simulink model "mtv1_with_slosh_with_valve_delay"  (R2014b)
settings: Solver=ode4  SolverMode=SingleTasking  StartTime=0.0  StopTime=sim_stop_time  FixedStep=sim_time_step_size  RelTol=1e-3
PreLoadFcn:
  | nimbus_bus_all;
  | mtv_bus_all;
undefined symbols (not defined in the file or in its folder): csc_cnt_attitude_control, csc_cnt_attitude_control_lib, csc_cnt_dt, csc_egt_egc_thruster, csc_egt_egc_thruster_lib, csc_eom_six_dof_integration_fwdeuler, csc_eom_six_dof_integration_lib, csc_ppc_phase_plane_ctrl, csc_ppc_phase_plane_ctrl_lib, csc_rigid_body_dynamics, csc_rigid_body_dynamics_lib, csc_sim_mtv_simulation, csc_sim_mtv_simulation_lib, csc_thl_thrusters_mtv, csc_thl_thrusters_mtv_lib, csci_fsw_mtv, csci_fsw_mtv_lib, csci_gsse_mtv, csci_gsse_mtv_lib, csu_rrk_rotational_kinematics, csu_rrk_rotational_kinematics_lib, csu_rtk_translational_kinematics, csu_rtk_translational_kinematics_lib, csu_tpl_thruster_propellant_mtv, csu_tpl_thruster_propellant_mtv_lib, egt_feed_pressure, egt_g_times_isp, egt_pc_to_thrust_offset, egt_pc_to_thrust_slope, gdn_altitude_transition_free_drift_landing, gdn_altitude_transition_free_drift_takeoff, ini_epoch_seconds, ini_landed_flag, ini_thrust_to_weight_takeoff_limit, mpl_gn2_mass_initial, mpl_htp_mass_initial, ppc_coarse_thr_delay, ppc_fine_thr_delay, sim_time_step_size, swm_num_switches, tpl_coarse_acs_thrust_to_isp, tpl_egc_chamber_pressure_to_thrust, tpl_egc_throttle_to_mdot_gain, tpl_egc_throttle_to_thrust, tpl_egc_throttle_to_thrust_gain
libraries: util_common_lib x17, util_info_lib x13, util_quat_lib x8, simulink x8, csu_spv_simulated_press_valves_lib x4, csu_cfe_cfe_time_lib x2, csu_tlm_telemetry_lib x2, util_event_lib x2, util_frame_rotation_lib x2, csc_act_actuator_manager_mtv_lib x1, csc_cmp_command_mode_process_mtv_lib x1, util_extra_lib x1
(part 1 of 2)
settings Model: ExtModeTrigDuration=100  Creator=ianmga  LastModifiedBy=mstewart
settings DataIOCC: LimitDataPoints=off  SaveOutput=off  SaveTime=off  StateSaveName=tmp_raccel_xout  SignalLoggingName=raw_event_logs
settings OptimizationCC: ExpressionDepthLimit=2147483647  InitFltsAndDblsToZero=on  OptimizeModelRefInitCode=on
settings DebuggingCC: CheckSSInitialOutputMsg=off  UnderspecifiedInitializationDetection=Classic  MergeDetectMultiDrivingBlocksExec=none  UnderSpecifiedDataTypeMsg=warning  FcnCallInpInsideContextMsg=UseLocalSettings  BusObjectLabelMismatch=error  StateNameClashWarn=warning  StrictBusMsg=WarnOnBusTreatedAsVector
settings HardwareCC: TargetHWDeviceType=32-bit Generic
settings SFSimCC: SimParseCustomCode=off
settings SFSimCC: SimUserIncludeDirs=|
  | ../sim/fhw/sensors/cameras/kir
  | ../fsw/est/kcv
  | ../fsw/est/kfd
  | ../externals/minopencv/include
settings RTWCC: SystemTargetFile=ert.tlc  GenCodeOnly=on  TemplateMakefile=ert_default_tmf  Description=Embedded Coder  RetainRTWFile=on  ProcessScript=ert_make_rtw_hook  RTWUseSimCustomCode=on
settings RTWCC: CustomInclude=|
  | ../sim/fhw/sensors/cameras/kir
  | ../fsw/est/kcv
  | ../fsw/est/kfd
  | ../externals/minopencv/include
settings CodeAppCC: ForceParamTrailComments=on  IgnoreCustomStorageClasses=off  MaxIdLength=128  SimulinkDataObjDesc=on  SFDataObjDesc=on  MangleLength=10  CustomSymbolStrType=$N$R$M  InsertBlockDesc=on  InternalIdentifier=Classic  ReqsInCode=on
settings ERTTargetCC: GenerateSampleERTMain=on  MultiInstanceERTCode=on  CodeInterfacePackaging=Reusable function  RootIOFormat=Structure reference  ERTCustomFileTemplate=csl_interface.tlc

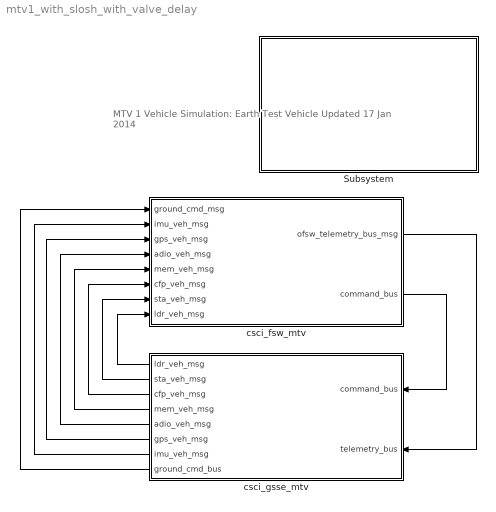
== system mtv1_with_slosh_with_valve_delay ==
  note: MTV 1 Vehicle Simulation: Earth Test Vehicle
      |
      | Updated 17 Jan 2014
  Subsystem : Subsystem
      mask Display: image('nimbus2.png')
  csci_fsw_mtv : Subsystem  AncestorBlock=csci_fsw_mtv_lib/csci_fsw_mtv
  csci_gsse_mtv : Subsystem  AncestorBlock=csci_gsse_mtv_lib/csci_gsse_mtv
  wires:
  csci_fsw_mtv/1(ofsw_telemetry_bus_msg) -> csci_gsse_mtv/2(telemetry_bus)
  csci_gsse_mtv/2(sta_veh_msg) -> csci_fsw_mtv/7(sta_veh_msg)
  csci_fsw_mtv/2(command_bus) -> csci_gsse_mtv/1(command_bus)
  csci_gsse_mtv/1(ldr_veh_msg) -> csci_fsw_mtv/8(ldr_veh_msg)
  csci_gsse_mtv/3(cfp_veh_msg) -> csci_fsw_mtv/6(cfp_veh_msg)
  csci_gsse_mtv/4(mem_veh_msg) -> csci_fsw_mtv/5(mem_veh_msg)
  csci_gsse_mtv/5(adio_veh_msg) -> csci_fsw_mtv/4(adio_veh_msg)
  csci_gsse_mtv/6(gps_veh_msg) -> csci_fsw_mtv/3(gps_veh_msg)
  csci_gsse_mtv/8(ground_cmd_bus) -> csci_fsw_mtv/1(ground_cmd_msg)
  csci_gsse_mtv/7(imu_veh_msg) -> csci_fsw_mtv/2(imu_veh_msg)

== system mtv1_with_slosh_with_valve_delay/Subsystem ==

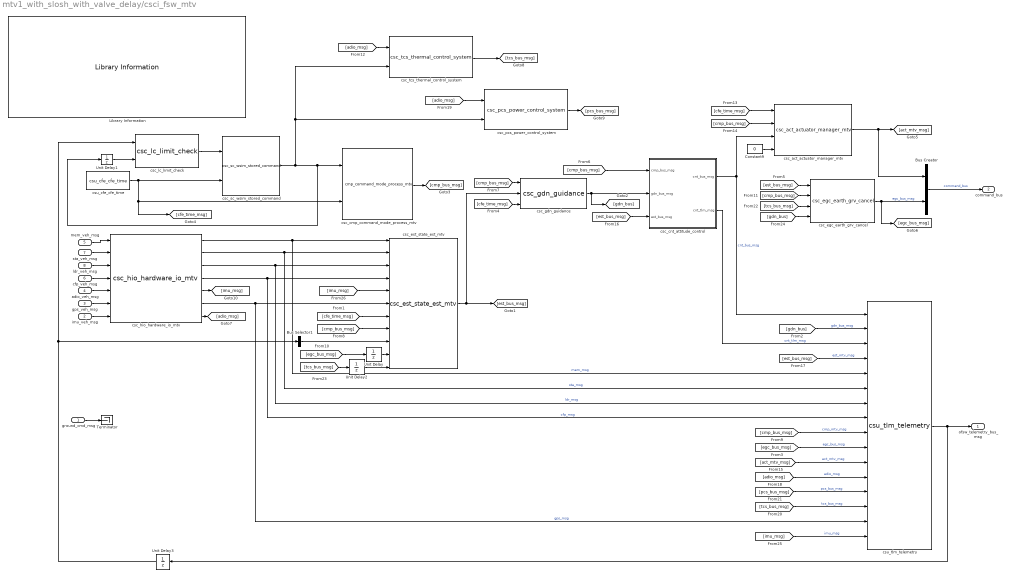
== system mtv1_with_slosh_with_valve_delay/csci_fsw_mtv ==
  ground_cmd_msg : Inport
  imu_veh_msg : Inport  Port=2
  gps_veh_msg : Inport  Port=3
  adio_veh_msg : Inport  Port=4
  mem_veh_msg : Inport  Port=5
  cfp_veh_msg : Inport  Port=6
  sta_veh_msg : Inport  Port=7
  ldr_veh_msg : Inport  Port=8
  Bus Creator : BusCreator  Inputs=2
  Bus Selector1 : BusSelector  OutputSignals=act_mtv_msg  OutputAsBus=on
  Constant9 : Constant  Value=0  OutDataTypeStr=uint32
  Library Information : util_info_lib/Library Information  owner='NONE'
  Terminator : Terminator
  Unit Delay{,1..3} (4 alike) : UnitDelay  SampleTime=-1
  csc_act_actuator_manager_mtv : csc_act_actuator_manager_mtv_lib/csc_act_actuator_manager_mtv  Tag=OFSW; MDL_TICK=CNT_BUS_MSG
  csc_cmp_command_mode_process_mtv : csc_cmp_command_mode_process_mtv_lib/cmp_command_mode_process_mtv  Tag=OFSW
  csc_cnt_attitude_control : Subsystem  Tag=OFSW; MDL_TICK=GDN_BUS_MSG  AncestorBlock=csc_cnt_attitude_control_lib/csc_cnt_attitude_control  TreatAsAtomicUnit=on  SystemSampleTime=csc_cnt_dt
  csc_egc_earth_grv_cancel : csc_egc_earth_grv_cancel_lib/csc_egc_earth_grv_cancel  Tag=OFSW; MDL_TICK=TCS_BUS_MSG
  csc_est_state_est_mtv : csc_est_state_est_mtv_lib/csc_est_state_est_mtv  Tag=OFSW; MDL_TICK=CMP_MTV_MSG
  csc_gdn_guidance : csc_gdn_guidance_lib/csc_gdn_guidance  Tag=OFSW; MDL_TICK=EST_MTV_MSG
  csc_hio_hardware_io_mtv : csc_hio_hardware_io_mv_lib/csc_hio_hardware_io_mtv
  csc_lc_limit_check : csc_lc_limit_check_lib/csc_lc_limit_check
  csc_pcs_power_control_system : csc_pcs_power_control_system_lib/csc_pcs_power_control_system  Tag=OFSW; MDL_TICK=ADIO_MSG
  csc_sc_wsim_stored_command : csc_sc_wsim_stored_command_lib/csc_sc_wsim_stored_command
  csc_tcs_thermal_control_system : csc_tcs_thermal_control_system_lib/csc_tcs_thermal_control_system  Tag=OFSW; MDL_TICK=ADIO_MSG
  csu_cfe_cfe_time : csu_cfe_cfe_time_lib/csu_cfe_cfe_time  sch_dt=fsw_dt
  csu_tlm_telemetry : csu_tlm_telemetry_lib/csu_tlm_telemetry  num_inputs=16  output_bus_name=ofsw_telemetry_bus_msg
  ofsw_telemetry_bus_msg : Outport
  command_bus : Outport  Port=2
  wires:
  [egc_bus_msg] -> Unit Delay/1
  [egc_bus_msg] -> csu_tlm_telemetry/10  "egc_bus_msg"
  csc_egc_earth_grv_cancel/1 -> Bus Creator/2, [egc_bus_msg]  "egc_bus_msg"
  [est_bus_msg] -> csc_egc_earth_grv_cancel/1
  Unit Delay1/1 -> csc_lc_limit_check/2
  Unit Delay3/1 -> csc_lc_limit_check/1, Bus Selector1/1
  csc_lc_limit_check/1 -> csc_sc_wsim_stored_command/1
  [cmp_bus_msg] -> csu_tlm_telemetry/9  "cmp_mtv_msg"
  csc_hio_hardware_io_mtv/4 -> csu_tlm_telemetry/8, csc_est_state_est_mtv/4  "cfp_msg"
  csc_hio_hardware_io_mtv/3 -> csu_tlm_telemetry/7, csc_est_state_est_mtv/3  "ldr_msg"
  csc_hio_hardware_io_mtv/2 -> csu_tlm_telemetry/6, csc_est_state_est_mtv/2  "sta_msg"
  cfp_veh_msg/1 -> csc_hio_hardware_io_mtv/4
  ldr_veh_msg/1 -> csc_hio_hardware_io_mtv/3
  sta_veh_msg/1 -> csc_hio_hardware_io_mtv/2
  csc_cnt_attitude_control/2(cnt_tlm_msg) -> csu_tlm_telemetry/3  "cnt_tlm_msg"
  [cmp_bus_msg] -> csc_gdn_guidance/1
  [cmp_bus_msg] -> csc_cnt_attitude_control/1(cmp_bus_msg)
  csc_cmp_command_mode_process_mtv/1 -> [cmp_bus_msg]
  csu_cfe_cfe_time/1 -> csc_cmp_command_mode_process_mtv/2, [cfe_time_msg], csc_sc_wsim_stored_command/2
  [cfe_time_msg] -> csc_gdn_guidance/3
  Bus Creator/1 -> command_bus/1  "command_bus"
  csu_tlm_telemetry/1 -> Unit Delay3/1, ofsw_telemetry_bus_msg/1
  ground_cmd_msg/1 -> Terminator/1
  csc_cnt_attitude_control/1(cnt_bus_msg) -> csc_act_actuator_manager_mtv/3, csu_tlm_telemetry/1  "cnt_bus_msg"
  csc_gdn_guidance/1 -> [gdn_bus], csc_cnt_attitude_control/2(gdn_bus_msg)
  csc_est_state_est_mtv/1 -> csc_gdn_guidance/2, [est_bus_msg]
  csc_sc_wsim_stored_command/1 -> csc_tcs_thermal_control_system/2, csc_pcs_power_control_system/2, Unit Delay1/1, csc_cmp_command_mode_process_mtv/1
  [cfe_time_msg] -> csc_est_state_est_mtv/7
  [cmp_bus_msg] -> csc_est_state_est_mtv/8
  Bus Selector1/1 -> csc_est_state_est_mtv/9
  Unit Delay/1 -> csc_est_state_est_mtv/10
  [gdn_bus] -> csu_tlm_telemetry/2  "gdn_bus_msg"
  csc_act_actuator_manager_mtv/1 -> [act_mtv_msg], Bus Creator/1
  [cfe_time_msg] -> csc_act_actuator_manager_mtv/1
  [cmp_bus_msg] -> csc_act_actuator_manager_mtv/2
  Constant9/1 -> csc_act_actuator_manager_mtv/4
  [act_mtv_msg] -> csu_tlm_telemetry/11  "act_mtv_msg"
  mem_veh_msg/1 -> csc_hio_hardware_io_mtv/1
  csc_hio_hardware_io_mtv/1 -> csu_tlm_telemetry/5, csc_est_state_est_mtv/1  "mem_msg"
  [est_bus_msg] -> csc_cnt_attitude_control/3(est_bus_msg)
  [est_bus_msg] -> csu_tlm_telemetry/4  "est_mtv_msg"
  [cmp_bus_msg] -> csc_egc_earth_grv_cancel/2
  adio_veh_msg/1 -> csc_hio_hardware_io_mtv/5
  csc_hio_hardware_io_mtv/7 -> [adio_msg]
  [adio_msg] -> csu_tlm_telemetry/12  "adio_msg"
  [adio_msg] -> csc_tcs_thermal_control_system/1
  [adio_msg] -> csc_pcs_power_control_system/1
  csc_tcs_thermal_control_system/1 -> [tcs_bus_msg]
  csc_pcs_power_control_system/1 -> [pcs_bus_msg]
  [pcs_bus_msg] -> csu_tlm_telemetry/13  "pcs_bus_msg"
  [tcs_bus_msg] -> csu_tlm_telemetry/14  "tcs_bus_msg"
  [tcs_bus_msg] -> csc_egc_earth_grv_cancel/3
  gps_veh_msg/1 -> csc_hio_hardware_io_mtv/6
  csc_hio_hardware_io_mtv/6 -> csu_tlm_telemetry/15, csc_est_state_est_mtv/6  "gps_msg"
  [tcs_bus_msg] -> Unit Delay2/1
  Unit Delay2/1 -> csc_est_state_est_mtv/11
  [gdn_bus] -> csc_egc_earth_grv_cancel/4
  imu_veh_msg/1 -> csc_hio_hardware_io_mtv/7
  csc_hio_hardware_io_mtv/5 -> [imu_msg]
  [imu_msg] -> csu_tlm_telemetry/16  "imu_msg"
  [imu_msg] -> csc_est_state_est_mtv/5

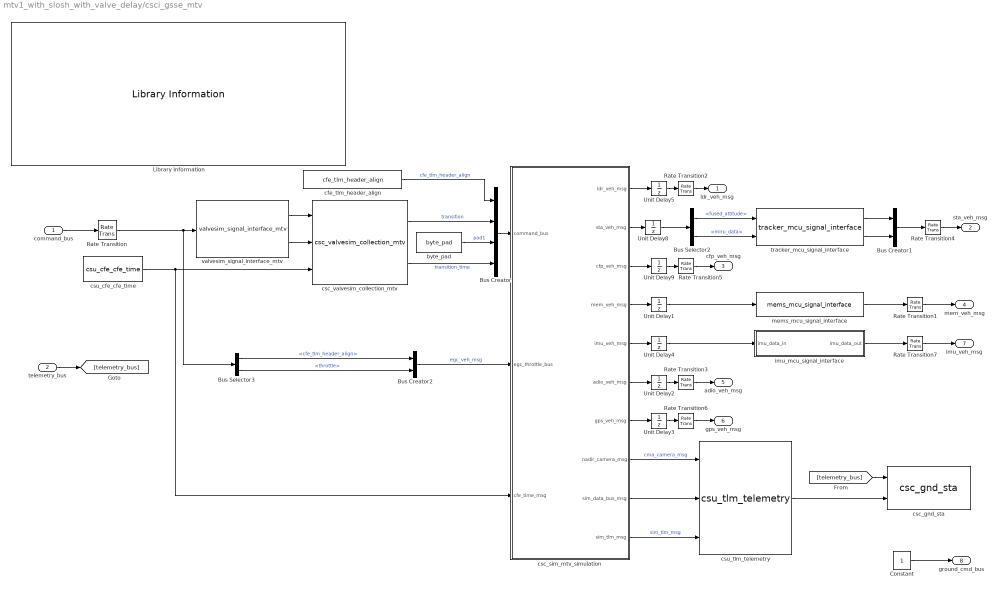
== system mtv1_with_slosh_with_valve_delay/csci_gsse_mtv ==
  command_bus : Inport
  telemetry_bus : Inport  Port=2
  Bus Creator : BusCreator  OutDataTypeStr=Bus: thr_sim_msg  NonVirtualBus=on
  Bus Creator2 : BusCreator  Inputs=2  OutDataTypeStr=Bus: egc_veh_msg  NonVirtualBus=on
  Bus Selector2 : BusSelector  OutputSignals=fused_attitude,miru_data
  Bus Selector3 : BusSelector  OutputSignals=egc_bus_msg.cfe_tlm_header_align,egc_bus_msg.throttle
  Bus Creator1 : BusCreator  Inputs=2
  Constant : Constant
  Library Information : util_info_lib/Library Information  owner='NONE'
  Rate Transition{,1..7} (8 alike) : RateTransition  Integrity=off
  Unit Delay{1..5,8..9} (7 alike) : UnitDelay  SampleTime=-1
  byte_pad : util_common_lib/byte_pad  n_bytes=6
  cfe_tlm_header_align : util_common_lib/cfe_tlm_header_align
  csc_gnd_sta : csc_gnd_sta_lib/csc_gnd_sta  dir_name=scenario_data_dir
  csc_sim_mtv_simulation : Subsystem  Tag=GSSE; MDL_TICK=THR_SIM_MSG  AncestorBlock=csc_sim_mtv_simulation_lib/csc_sim_mtv_simulation  TreatAsAtomicUnit=on
  csc_valvesim_collection_mtv : csc_valvesim_collection_mtv_lib/csc_valvesim_collection_mtv  SystemSampleTime=-1
  csu_cfe_cfe_time : csu_cfe_cfe_time_lib/csu_cfe_cfe_time  sch_dt=sim_time_step_size
  csu_tlm_telemetry : csu_tlm_telemetry_lib/csu_tlm_telemetry  num_inputs=3  output_bus_name=sim_telemetry_bus_msg
  imu_mcu_signal_interface : Subsystem
  mems_mcu_signal_interface : csu_mems_mcu_signal_interface_lib/mems_mcu_signal_interface
  tracker_mcu_signal_interface : csu_tracker_mcu_signal_interface_lib/tracker_mcu_signal_interface
  valvesim_signal_interface_mtv : csu_valvesim_signal_interface_mtv_lib/valvesim_signal_interface_mtv
  ldr_veh_msg : Outport
  sta_veh_msg : Outport  Port=2
  cfp_veh_msg : Outport  Port=3
  mem_veh_msg : Outport  Port=4
  adio_veh_msg : Outport  Port=5
  gps_veh_msg : Outport  Port=6
  imu_veh_msg : Outport  Port=7
  ground_cmd_bus : Outport  Port=8
  wires:
  telemetry_bus/1 -> [telemetry_bus]
  csc_sim_mtv_simulation/9(sim_data_bus_msg) -> csu_tlm_telemetry/2
  Unit Delay9/1 -> Rate Transition5/1
  Unit Delay5/1 -> Rate Transition2/1
  csc_sim_mtv_simulation/1(ldr_veh_msg) -> Unit Delay5/1
  csc_sim_mtv_simulation/3(cfp_veh_msg) -> Unit Delay9/1
  Constant/1 -> ground_cmd_bus/1
  command_bus/1 -> Rate Transition/1
  Rate Transition2/1 -> ldr_veh_msg/1
  Rate Transition4/1 -> sta_veh_msg/1
  Rate Transition5/1 -> cfp_veh_msg/1
  csc_sim_mtv_simulation/2(sta_veh_msg) -> Unit Delay8/1
  csc_sim_mtv_simulation/8(nadir_camera_msg) -> csu_tlm_telemetry/1  "cma_camera_msg"
  csc_sim_mtv_simulation/10(sim_tlm_msg) -> csu_tlm_telemetry/3  "sim_tlm_msg"
  csu_tlm_telemetry/1 -> csc_gnd_sta/2
  [telemetry_bus] -> csc_gnd_sta/1
  valvesim_signal_interface_mtv/1 -> csc_valvesim_collection_mtv/1
  csc_valvesim_collection_mtv/1 -> Bus Creator/2  "transition"
  csc_valvesim_collection_mtv/2 -> Bus Creator/4  "transition_time"
  Bus Creator/1 -> csc_sim_mtv_simulation/1(command_bus)
  csu_cfe_cfe_time/1 -> csc_sim_mtv_simulation/3(cfe_time_msg), csc_valvesim_collection_mtv/3
  byte_pad/1 -> Bus Creator/3  "pad1"
  Rate Transition/1 -> Bus Selector3/1, valvesim_signal_interface_mtv/1
  Bus Creator2/1 -> csc_sim_mtv_simulation/2(egc_throttle_bus)  "egc_veh_msg"
  cfe_tlm_header_align/1 -> Bus Creator/1  "cfe_tlm_header_align"
  valvesim_signal_interface_mtv/2 -> csc_valvesim_collection_mtv/2
  Bus Creator1/1 -> Rate Transition4/1
  tracker_mcu_signal_interface/2 -> Bus Creator1/2
  tracker_mcu_signal_interface/1 -> Bus Creator1/1
  Bus Selector2/2 -> tracker_mcu_signal_interface/2  "<miru_data>"
  Bus Selector2/1 -> tracker_mcu_signal_interface/1  "<fused_attitude>"
  Unit Delay8/1 -> Bus Selector2/1
  csc_sim_mtv_simulation/4(mem_veh_msg) -> Unit Delay1/1
  Unit Delay1/1 -> mems_mcu_signal_interface/1
  Rate Transition1/1 -> mem_veh_msg/1
  mems_mcu_signal_interface/1 -> Rate Transition1/1
  Bus Selector3/1 -> Bus Creator2/1  "<cfe_tlm_header_align>"
  Bus Selector3/2 -> Bus Creator2/2  "<throttle>"
  Unit Delay2/1 -> Rate Transition3/1
  csc_sim_mtv_simulation/6(adio_veh_msg) -> Unit Delay2/1
  Rate Transition3/1 -> adio_veh_msg/1
  Unit Delay3/1 -> Rate Transition6/1
  Rate Transition6/1 -> gps_veh_msg/1
  csc_sim_mtv_simulation/7(gps_veh_msg) -> Unit Delay3/1
  csc_sim_mtv_simulation/5(imu_veh_msg) -> Unit Delay4/1
  Unit Delay4/1 -> imu_mcu_signal_interface/1(imu_data_in)
  Rate Transition7/1 -> imu_veh_msg/1
  imu_mcu_signal_interface/1(imu_data_out) -> Rate Transition7/1

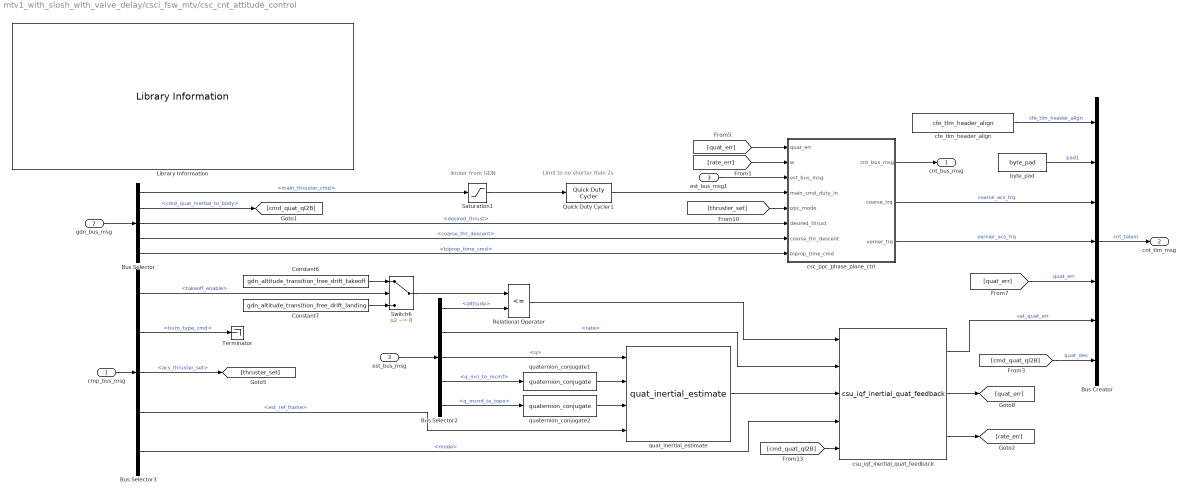
== system mtv1_with_slosh_with_valve_delay/csci_fsw_mtv/csc_cnt_attitude_control ==
  note: Limit to no shorter than 2s
  note: limiter from GDN
  cmp_bus_msg : Inport
  gdn_bus_msg : Inport  Port=2  OutDataTypeStr=Bus: gdn_bus_msg
  est_bus_msg : Inport  Port=3
  Bus Creator : BusCreator  Inputs=7  OutDataTypeStr=Bus: cnt_tlm_msg  NonVirtualBus=on
  Bus Selector2 : BusSelector  OutputSignals=altitude,rate,q,q_mci_to_mcmf,q_mcmf_to_topo
  Bus Selector3 : BusSelector  OutputSignals=takeoff_enable,burn_type_cmd,acs_thruster_set,est_ref_frame,mode
  Bus Selector : BusSelector  OutputSignals=main_thruster_cmd,cmd_quat_inertial_to_body,desired_thrust,coarse_thr_descent,biprop_time_cmd
  Constant6 : Constant  Value=gdn_altitude_transition_free_drift_takeoff  VectorParams1D=off
  Constant7 : Constant  Value=gdn_altitude_transition_free_drift_landing  VectorParams1D=off
  Library Information : util_info_lib/Library Information  owner='NONE'
  Quick Duty Cycler1 : util_extra_lib/Quick Duty Cycler  min_dt=2  dt=csc_cnt_dt
  Relational Operator : RelationalOperator  Operator=<=  OutDataTypeStr=boolean
  Saturation1 : Saturate  UpperLimit=1.1  LowerLimit=0.0
  Switch6 : Switch  Criteria=u2 ~= 0
  Terminator : Terminator
  byte_pad : util_common_lib/byte_pad  n_bytes=6
  cfe_tlm_header_align : util_common_lib/cfe_tlm_header_align
  csc_ppc_phase_plane_ctrl : Subsystem  AncestorBlock=csc_ppc_phase_plane_ctrl_lib/csc_ppc_phase_plane_ctrl
  csu_iqf_inertial_quat_feedback : csu_iqf_inertial_quat_feedback_lib/csu_iqf_inertial_quat_feedback
  est_bus_msg1 : InportShadow  Port=3
  quat_inertial_estimate : util_quat_lib/quat_inertial_estimate  SystemSampleTime=-1
  quaternion_conjugate1 : util_quat_lib/quaternion_conjugate  SystemSampleTime=-1
  quaternion_conjugate2 : util_quat_lib/quaternion_conjugate  SystemSampleTime=-1
  cnt_bus_msg : Outport  OutDataTypeStr=Bus: cnt_bus_msg
  cnt_tlm_msg : Outport  Port=2  OutDataTypeStr=Bus: cnt_tlm_msg
  wires:
  Bus Selector/5 -> csc_ppc_phase_plane_ctrl/8(biprop_time_cmd)  "<biprop_time_cmd>"
  Bus Selector/3 -> csc_ppc_phase_plane_ctrl/6(desired_thrust)  "<desired_thrust>"
  byte_pad/1 -> Bus Creator/2  "pad1"
  Quick Duty Cycler1/1 -> csc_ppc_phase_plane_ctrl/4(main_cmd_duty_in)
  csc_ppc_phase_plane_ctrl/1(cnt_bus_msg) -> cnt_bus_msg/1
  csu_iqf_inertial_quat_feedback/2 -> [quat_err]
  Constant6/1 -> Switch6/1
  Constant7/1 -> Switch6/3
  cmp_bus_msg/1 -> Bus Selector3/1
  Bus Selector3/1 -> Switch6/2  "<takeoff_enable>"
  [quat_err] -> Bus Creator/5  "quat_err"
  gdn_bus_msg/1 -> Bus Selector/1
  Bus Creator/1 -> cnt_tlm_msg/1  "cnt_telem"
  Bus Selector/2 -> [cmd_quat_qI2B]  "<cmd_quat_inertial_to_body>"
  [cmd_quat_qI2B] -> Bus Creator/7  "quat_des"
  Bus Selector/1 -> Saturation1/1  "<main_thruster_cmd>"
  Bus Selector3/2 -> Terminator/1  "<burn_type_cmd>"
  est_bus_msg/1 -> Bus Selector2/1
  Bus Selector2/3 -> quat_inertial_estimate/1  "<q>"
  [cmd_quat_qI2B] -> csu_iqf_inertial_quat_feedback/5
  [quat_err] -> csc_ppc_phase_plane_ctrl/1(quat_err)
  Bus Selector3/3 -> [thruster_set]  "<acs_thruster_set>"
  [thruster_set] -> csc_ppc_phase_plane_ctrl/5(ppc_mode)
  Bus Selector/4 -> csc_ppc_phase_plane_ctrl/7(coarse_thr_descent)  "<coarse_thr_descent>"
  Switch6/1 -> Relational Operator/1
  est_bus_msg1/1 -> csc_ppc_phase_plane_ctrl/3(est_bus_msg)
  Bus Selector3/5 -> csu_iqf_inertial_quat_feedback/4  "<mode>"
  Saturation1/1 -> Quick Duty Cycler1/1
  csc_ppc_phase_plane_ctrl/2(coarse_trq) -> Bus Creator/3  "coarse_acs_trq"
  csc_ppc_phase_plane_ctrl/3(verner_trq) -> Bus Creator/4  "vernier_acs_trq"
  quat_inertial_estimate/1 -> csu_iqf_inertial_quat_feedback/3
  Bus Selector2/4 -> quaternion_conjugate1/1  "<q_mci_to_mcmf>"
  Bus Selector2/5 -> quaternion_conjugate2/1  "<q_mcmf_to_topo>"
  Bus Selector2/1 -> Relational Operator/2  "<altitude>"
  Bus Selector3/4 -> quat_inertial_estimate/4  "<est_ref_frame>"
  csu_iqf_inertial_quat_feedback/1 -> Bus Creator/6  "sat_quat_err"
  Relational Operator/1 -> csu_iqf_inertial_quat_feedback/1
  quaternion_conjugate1/1 -> quat_inertial_estimate/2
  quaternion_conjugate2/1 -> quat_inertial_estimate/3
  cfe_tlm_header_align/1 -> Bus Creator/1  "cfe_tlm_header_align"
  Bus Selector2/2 -> csu_iqf_inertial_quat_feedback/2  "<rate>"
  csu_iqf_inertial_quat_feedback/3 -> [rate_err]
  [rate_err] -> csc_ppc_phase_plane_ctrl/2(w)

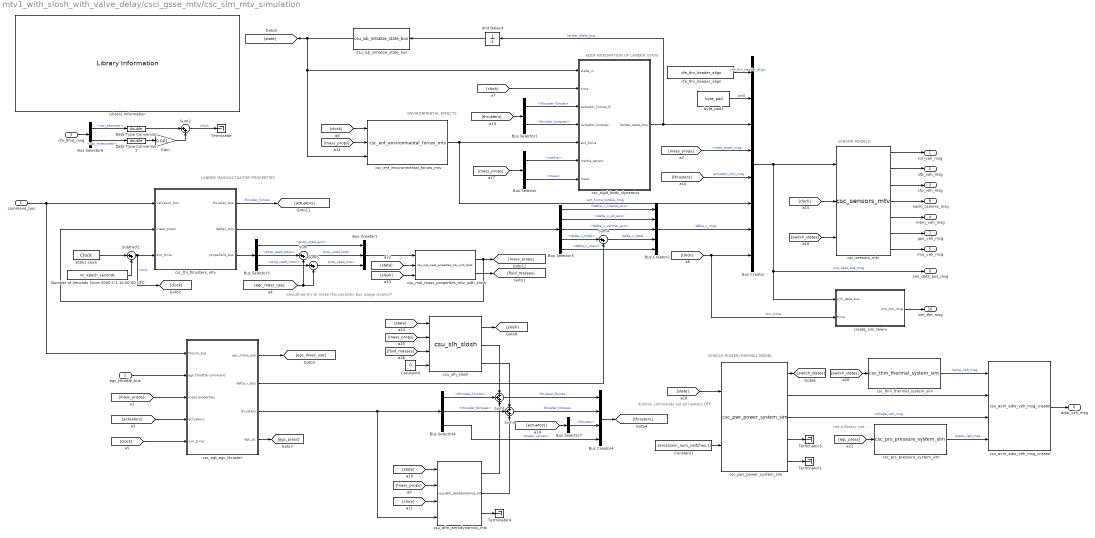
== system mtv1_with_slosh_with_valve_delay/csci_gsse_mtv/csc_sim_mtv_simulation ==
  note: not a library yet....
  note: VEHICLE POWER/THERMAL MODEL
  note: dummy commands set all heaters OFF
  note: LANDER MASS/ACTUATOR PROPERTIES
  note: 6DOF INTEGRATION OF LANDER STATE
  note: ENVIRONMENTAL EFFECTS
  note: SENSOR MODELS
  note: Should we try to make this parasitic bus usage cleaner?
  command_bus : Inport
  egc_throttle_bus : Inport  Port=2
  cfe_time_msg : Inport  Port=3  OutDataTypeStr=Bus: cfe_time_msg
  100hz clock : DigitalClock  SampleTime=sim_time_step_size
  Bus Creator : BusCreator  Inputs=8  OutDataTypeStr=Bus: sim_data_mtv_msg  NonVirtualBus=on
  Bus Creator1 : BusCreator  Inputs=3
  Bus Creator2 : BusCreator  Inputs=5
  Bus Creator4 : BusCreator  OutDataTypeStr=Bus: actuator_mtv_msg_t
  Bus Selector : BusSelector  OutputSignals=inertia,mass
  Bus Selector1 : BusSelector  OutputSignals=thruster_forces,thruster_torques
  Bus Selector3 : BusSelector  OutputSignals=prop_used_acs,prop_used_total,prop_used_main
  Bus Selector4 : BusSelector  OutputSignals=thruster_forces,thruster_torques,press_valves
  Bus Selector5 : BusSelector  OutputSignals=delta_v_coarse_acs,delta_v_all_acs,delta_v_vernier_acs,delta_v_total,delta_v_main
  Bus Selector6 : BusSelector  OutputSignals=utc_seconds,utc_mseconds
  Bus Selector7 : BusSelector  OutputSignals=thrusts
  Constant1 : Constant  Value=zeros(swm_num_switches,1)  OutDataTypeStr=double
  Constant4 : Constant  Value=0
  Data Type Conversion : DataTypeConversion  OutDataTypeStr=double
  Data Type Conversion1 : DataTypeConversion  OutDataTypeStr=double
  Gain : Gain  Gain=0.001
  Library Information : util_info_lib/Library Information  owner='NONE'
  Number of Seconds Since 2000-1-1 12:00:00 UTC : Constant  Description=|  Value=ini_epoch_seconds
      | Number of Seconds                   
      | July 4, 2014 22:40:00 UTC           
      | Calculate on Web Site:              
      | www.mbari.org/staff/rich/utccalc.htm
  Subtract1 : Sum  Inputs=|++
  Sum{,2,4..5} (4 alike) : Sum  Inputs=|++
  Sum1 : Sum  Inputs=+++
  Sum3 : Sum  Inputs=+++
  Terminator{,1,3..4} (4 alike) : Terminator
  Unit Delay4 : UnitDelay  SampleTime=-1
  byte_pad1 : util_common_lib/byte_pad  n_bytes=4
  cfe_tlm_header_align : util_common_lib/cfe_tlm_header_align
  create_sim_telem : Subsystem
  csc_egt_egc_thruster : Subsystem  AncestorBlock=csc_egt_egc_thruster_lib/csc_egt_egc_thruster
  csc_enf_environmental_forces_mtv : csc_enf_environmental_forces_mtv_lib/csc_enf_environmental_forces_mtv
  csc_prs_pressure_system_sim : csc_prs_pressure_system_sim_lib/csc_prs_pressure_system_sim
  csc_pwr_power_system_sim : csc_pwr_power_system_sim_lib/csc_pwr_power_system_sim
  csc_rigid_body_dynamics : Subsystem  AncestorBlock=csc_rigid_body_dynamics_lib/csc_rigid_body_dynamics
  csc_sensors_mtv : csc_sensors_mtv_lib/csc_sensors_mtv
  csc_thl_thrusters_mtv : Subsystem  AncestorBlock=csc_thl_thrusters_mtv_lib/csc_thl_thrusters_mtv
  csc_thm_thermal_system_sim : csc_thm_thermal_system_sim_lib/csc_thm_thermal_system_sim
  csu_afm_aerodynamics_mtv : csu_afm_aerodynamics_lib/csu_afm_aerodynamics_mtv  SystemSampleTime=-1
  csu_avm_adio_veh_msg_creator : csu_avm_adio_veh_msg_creator_lib/csu_avm_adio_veh_msg_creator
  csu_isb_initialize_state_bus : csu_isb_initialize_state_bus_lib/csu_isb_initialize_state_bus
  csu_mpl_mass_properties_mtv_with_slosh : csu_mpl_mass_properties_mtv_lib/csu_mpl_mass_properties_mtv_with_slosh
  csu_slh_slosh : csu_slh_slosh/csu_slh_slosh
  ldr_veh_msg : Outport
  sta_veh_msg : Outport  Port=2
  cfp_veh_msg : Outport  Port=3
  mem_veh_msg : Outport  Port=4
  imu_veh_msg : Outport  Port=5
  adio_veh_msg : Outport  Port=6
  gps_veh_msg : Outport  Port=7
  nadir_camera_msg : Outport  Port=8
  sim_data_bus_msg : Outport  Port=9
  sim_tlm_msg : Outport  Port=10
  wires:
  csu_afm_aerodynamics_mtv/3 -> Terminator4/1
  [clock] -> csu_afm_aerodynamics_mtv/3
  csu_afm_aerodynamics_mtv/2 -> Sum3/3
  Sum3/1 -> Bus Creator4/2  "thruster_torques"
  csu_afm_aerodynamics_mtv/1 -> Sum1/3
  Bus Selector7/1 -> Bus Creator4/3  "<thrusts>"
  [actuators] -> Bus Selector7/1
  Bus Creator4/1 -> [thrusters]
  Sum1/1 -> Bus Creator4/1  "thruster_forces"
  Bus Selector4/1 -> Sum1/2  "<thruster_forces>"
  Bus Selector4/2 -> Sum3/2  "<thruster_torques>"
  csc_egt_egc_thruster/3(thrusters) -> csu_afm_aerodynamics_mtv/4, Bus Selector4/1
  [switch_states] -> csc_sensors_mtv/3
  csc_pwr_power_system_sim/5 -> Terminator1/1
  csc_pwr_power_system_sim/4 -> Terminator3/1
  csc_pwr_power_system_sim/1 -> [switch_states]
  [state] -> csc_pwr_power_system_sim/1
  Constant1/1 -> csc_pwr_power_system_sim/2
  [clock] -> csc_sensors_mtv/2
  Unit Delay4/1 -> csu_isb_initialize_state_bus/1
  csu_isb_initialize_state_bus/1 -> csc_enf_environmental_forces_mtv/3, csc_rigid_body_dynamics/1(state_in), [state]
  [clock] -> csc_rigid_body_dynamics/2(time)
  cfe_tlm_header_align/1 -> Bus Creator/1  "cfe_tlm_header_align"
  csc_sensors_mtv/4 -> nadir_camera_msg/1
  csc_sensors_mtv/3 -> cfp_veh_msg/1
  csc_sensors_mtv/2 -> sta_veh_msg/1
  csc_sensors_mtv/1 -> ldr_veh_msg/1
  Bus Selector6/1 -> Data Type Conversion/1  "<utc_seconds>"
  Gain/1 -> Sum2/2
  Data Type Conversion1/1 -> Gain/1
  Data Type Conversion/1 -> Sum2/1
  Bus Selector6/2 -> Data Type Conversion1/1  "<utc_mseconds>"
  cfe_time_msg/1 -> Bus Selector6/1
  egc_throttle_bus/1 -> csc_egt_egc_thruster/2(egc throttle command)
  [mass_props] -> csc_egt_egc_thruster/3(mass properties)
  [actuators] -> csc_egt_egc_thruster/4(actuators)
  Bus Selector5/1 -> Bus Creator2/1  "<delta_v_coarse_acs>"
  Bus Selector5/2 -> Bus Creator2/2  "<delta_v_all_acs>"
  Bus Selector5/3 -> Bus Creator2/3  "<delta_v_vernier_acs>"
  Bus Selector5/5 -> Bus Creator2/5  "<delta_v_main>"
  Sum4/1 -> Bus Creator2/4  "delta_v_total"
  Bus Selector5/4 -> Sum4/1  "<delta_v_total>"
  csc_thl_thrusters_mtv/2(deltav_bus) -> Bus Selector5/1
  Bus Creator2/1 -> Bus Creator/7  "delta_v_msg"
  csc_egt_egc_thruster/2(delta_v_bus) -> Sum4/2
  Bus Selector3/3 -> Sum5/1  "<prop_used_main>"
  Bus Selector3/1 -> Bus Creator1/1  "<prop_used_acs>"
  Sum/1 -> Bus Creator1/2  "prop_used_total"
  [egc_mass_use] -> Sum5/2, Sum/2
  Bus Selector3/2 -> Sum/1  "<prop_used_total>"
  csc_egt_egc_thruster/1(egc_mass_use) -> [egc_mass_use]
  csc_thl_thrusters_mtv/3(propellant_bus) -> Bus Selector3/1
  byte_pad1/1 -> Bus Creator/2  "pad1"
  Subtract1/1 -> [clock], csc_thl_thrusters_mtv/3(sim_time)  "clock"
  [clock] -> Bus Creator/8, create_sim_telem/2(time)  "sim_time"
  create_sim_telem/1(sim_tlm_msg) -> sim_tlm_msg/1
  Bus Creator/1 -> create_sim_telem/1(sim_data_bus), sim_data_bus_msg/1, csc_sensors_mtv/1  "sim_data_bus_msg"
  csc_rigid_body_dynamics/1(lander_state_bus) -> Unit Delay4/1, Bus Creator/3  "lander_state_bus"
  [mass_props] -> Bus Selector/1
  [thrusters] -> Bus Selector1/1
  [thrusters] -> Bus Creator/5  "actuator_mtv_msg"
  [mass_props] -> Bus Creator/4  "mass_props_msg"
  Bus Selector/2 -> csc_rigid_body_dynamics/7(mass)  "<mass>"
  Bus Selector/1 -> csc_rigid_body_dynamics/6(inertia_tensor)  "<inertia>"
  Bus Selector1/1 -> csc_rigid_body_dynamics/3(actuator_forces_B)  "<thruster_forces>"
  Bus Selector1/2 -> csc_rigid_body_dynamics/4(actuator_torques)  "<thruster_torques>"
  csc_enf_environmental_forces_mtv/1 -> csc_rigid_body_dynamics/5(ext_force), Bus Creator/6  "enf_force_torque_msg"
  csc_thl_thrusters_mtv/1(thruster_bus) -> [actuators]  "thruster_forces"
  [clock] -> csc_enf_environmental_forces_mtv/1
  [mass_props] -> csc_enf_environmental_forces_mtv/2
  csc_sensors_mtv/5 -> mem_veh_msg/1
  Number of Seconds Since 2000-1-1 12:00:00 UTC/1 -> Subtract1/2
  100hz clock/1 -> Subtract1/1
  Sum2/1 -> Terminator/1  "clock"
  [switch_states] -> csc_thm_thermal_system_sim/1
  csu_avm_adio_veh_msg_creator/1 -> adio_veh_msg/1
  csc_thm_thermal_system_sim/1 -> csu_avm_adio_veh_msg_creator/1  "temp_veh_msg"
  csc_pwr_power_system_sim/2 -> csu_avm_adio_veh_msg_creator/2
  csc_pwr_power_system_sim/3 -> csu_avm_adio_veh_msg_creator/3  "voltage_veh_msg"
  [egc_press] -> csc_prs_pressure_system_sim/1
  csc_prs_pressure_system_sim/1 -> csu_avm_adio_veh_msg_creator/4  "press_veh_msg"
  csc_egt_egc_thruster/4(egc_pc) -> [egc_press]
  command_bus/1 -> csc_egt_egc_thruster/1(thrsim_bus), csc_thl_thrusters_mtv/1(valvesim_bus)
  [clock] -> csc_egt_egc_thruster/5(sim_time)
  Sum5/1 -> Bus Creator1/3  "prop_used_main"
  Bus Selector4/3 -> Bus Creator4/4  "<press_valves>"
  csc_sensors_mtv/6 -> gps_veh_msg/1
  csc_sensors_mtv/7 -> imu_veh_msg/1
  [mass_props] -> csu_afm_aerodynamics_mtv/2
  [state] -> csu_afm_aerodynamics_mtv/1
  Bus Creator1/1 -> csu_mpl_mass_properties_mtv_with_slosh/1
  csu_mpl_mass_properties_mtv_with_slosh/1 -> [mass_props], csc_thl_thrusters_mtv/2(mass_props)
  csu_mpl_mass_properties_mtv_with_slosh/2 -> [fluid_masses]
  [state] -> csu_mpl_mass_properties_mtv_with_slosh/2
  [state] -> csu_slh_slosh/1
  [mass_props] -> csu_slh_slosh/2
  [fluid_masses] -> csu_slh_slosh/3
  Constant4/1 -> csu_slh_slosh/4
  csu_slh_slosh/3 -> Sum3/1
  csu_slh_slosh/2 -> Sum1/1
  csu_slh_slosh/1 -> [slosh]
  [slosh] -> csu_mpl_mass_properties_mtv_with_slosh/3

== system mtv1_with_slosh_with_valve_delay/csci_gsse_mtv/imu_mcu_signal_interface ==
  imu_data_in : Inport
  Bus Selector2 : BusSelector  OutputSignals=cfe_tlm_header_align,gyro,accel,incline
  Bus Creator1 : BusCreator  Inputs=7
  Constant1 : Constant  Value=0  OutDataTypeStr=uint8
  Constant3 : Constant  OutDataTypeStr=uint16
  Constant4 : Constant  OutDataTypeStr=uint8
  Memory1 : Memory  X0=zeros(10,3)  InheritSampleTime=on
  Memory2 : Memory  X0=zeros(10,3)  InheritSampleTime=on
  Memory9 : Memory  X0=zeros(10,3)  InheritSampleTime=on
  Reshape1 : Reshape  OutputDimensionality=Row vector (2-D)
  Reshape2 : Reshape  OutputDimensionality=Row vector (2-D)
  Reshape9 : Reshape  OutputDimensionality=Row vector (2-D)
  Selector1 : Selector  NumberOfDimensions=2  InputPortWidth=10  IndexOptions=Index vector (dialog),Select all  Indices=[1:9],1  OutputSizes=1,1
  Selector2 : Selector  NumberOfDimensions=2  InputPortWidth=10  IndexOptions=Index vector (dialog),Select all  Indices=[1:9],1  OutputSizes=1,1
  Selector3 : Selector  NumberOfDimensions=2  InputPortWidth=10  IndexOptions=Index vector (dialog),Select all  Indices=[1:9],1  OutputSizes=1,1
  Vector Concatenate1 : Concatenate  Mode=Multidimensional array
  Vector Concatenate2 : Concatenate  Mode=Multidimensional array
  Vector Concatenate9 : Concatenate  Mode=Multidimensional array
  imu_data_out : Outport
  wires:
  Bus Selector2/4 -> Reshape1/1  "<incline>"
  Memory2/1 -> Selector3/1
  Selector3/1 -> Vector Concatenate2/2
  Vector Concatenate2/1 -> Bus Creator1/4, Memory2/1  "incline"
  Reshape1/1 -> Vector Concatenate2/1
  Bus Selector2/1 -> Bus Creator1/1  "<cfe_tlm_header_align>"
  Bus Creator1/1 -> imu_data_out/1  "imu_packet_data"
  imu_data_in/1 -> Bus Selector2/1
  Memory1/1 -> Selector1/1
  Selector1/1 -> Vector Concatenate1/2
  Vector Concatenate1/1 -> Memory1/1, Bus Creator1/2  "gyro"
  Reshape2/1 -> Vector Concatenate1/1
  Memory9/1 -> Selector2/1
  Selector2/1 -> Vector Concatenate9/2
  Vector Concatenate9/1 -> Bus Creator1/3, Memory9/1  "accel"
  Reshape9/1 -> Vector Concatenate9/1
  Constant3/1 -> Bus Creator1/5  "valid"
  Constant4/1 -> Bus Creator1/6  "active"
  Constant1/1 -> Bus Creator1/7  "mcu_fault"
  Bus Selector2/2 -> Reshape2/1  "<gyro>"
  Bus Selector2/3 -> Reshape9/1  "<accel>"

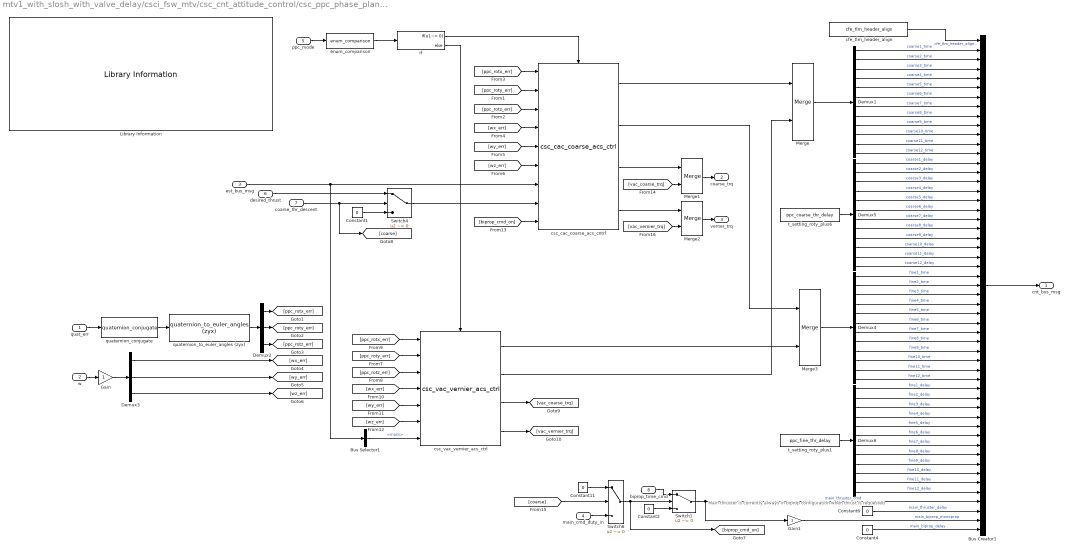
== system mtv1_with_slosh_with_valve_delay/csci_fsw_mtv/csc_cnt_attitude_control/csc_ppc_phase_plane_ctrl ==
  note: Main thruster is currently always in biprop configuration
      | when thrust is requested
  quat_err : Inport
  w : Inport  Port=2
  est_bus_msg : Inport  Port=3
  main_cmd_duty_in : Inport  Port=4
  ppc_mode : Inport  Port=5
  desired_thrust : Inport  Port=6
  coarse_thr_descent : Inport  Port=7
  biprop_time_cmd : Inport  Port=8
  Bus Creator1 : BusCreator  Inputs=53  OutDataTypeStr=Bus: cnt_bus_msg  NonVirtualBus=on
  Bus Selector1 : BusSelector  OutputSignals=mass
  Constant1 : Constant  Value=0
  Constant11 : Constant  Value=0  OutDataTypeStr=boolean
  Constant2 : Constant  Value=0  OutDataTypeStr=uint8
  Constant4 : Constant  Value=0  OutDataTypeStr=uint8
  Constant6 : Constant  Value=0  OutDataTypeStr=uint8
  Demux{1,4..6} (4 alike) : Demux  Outputs=12
  Demux2 : Demux  Outputs=3
  Demux3 : Demux  Outputs=3
  Gain : Gain
  Gain1 : Gain  OutDataTypeStr=uint8
  If : If  IfExpression=u1~= 0
  Library Information : util_info_lib/Library Information  owner='jkaidy'
  Merge{,1..3} (4 alike) : Merge
  Switch1 : Switch  Criteria=u2 ~= 0
  Switch4 : Switch  Criteria=u2 ~= 0
  Switch6 : Switch  Criteria=u2 ~= 0
  cfe_tlm_header_align : util_common_lib/cfe_tlm_header_align
  csc_cac_coarse_acs_cntrl : csc_cac_coarse_acs_ctrl_lib/csc_cac_coarse_acs_ctrl
  csc_vac_vernier_acs_ctrl : csc_vac_vernier_acs_ctrl_lib/csc_vac_vernier_acs_ctrl
  enum_comparison : util_common_lib/enum_comparison  comparison_type===
  quaternion_conjugate : util_quat_lib/quaternion_conjugate  SystemSampleTime=-1
  quaternion_to_euler_angles (zyx) : util_quat_lib/quaternion_to_euler_angles (zyx)  SystemSampleTime=-1
  t_setting_roty_plus1 : Constant  Value=ppc_fine_thr_delay  OutDataTypeStr=uint8
  t_setting_roty_plus6 : Constant  Value=ppc_coarse_thr_delay  OutDataTypeStr=uint8
  cnt_bus_msg : Outport
  coarse_trq : Outport  Port=2
  verner_trq : Outport  Port=3
  wires:
  [biprop_cmd_on] -> csc_cac_coarse_acs_cntrl/9
  Bus Selector1/1 -> csc_vac_vernier_acs_ctrl/7  "<mass>"
  csc_cac_coarse_acs_cntrl/1 -> Merge/1
  Demux3/3 -> [wz_err]
  Demux3/2 -> [wy_err]
  Demux3/1 -> [wx_err]
  Gain/1 -> Demux3/1
  est_bus_msg/1 -> csc_cac_coarse_acs_cntrl/7, Bus Selector1/1
  ppc_mode/1 -> enum_comparison/1
  [ppc_rotx_err] -> csc_vac_vernier_acs_ctrl/1
  [ppc_roty_err] -> csc_vac_vernier_acs_ctrl/2
  [ppc_rotz_err] -> csc_vac_vernier_acs_ctrl/3
  [wz_err] -> csc_vac_vernier_acs_ctrl/6
  [wx_err] -> csc_vac_vernier_acs_ctrl/4
  [wy_err] -> csc_vac_vernier_acs_ctrl/5
  [wz_err] -> csc_cac_coarse_acs_cntrl/6
  [ppc_roty_err] -> csc_cac_coarse_acs_cntrl/2
  [ppc_rotx_err] -> csc_cac_coarse_acs_cntrl/1
  [wx_err] -> csc_cac_coarse_acs_cntrl/4
  [wy_err] -> csc_cac_coarse_acs_cntrl/5
  [ppc_rotz_err] -> csc_cac_coarse_acs_cntrl/3
  w/1 -> Gain/1
  quat_err/1 -> quaternion_conjugate/1
  biprop_time_cmd/1 -> Switch1/1
  Constant2/1 -> Switch1/3
  [coarse] -> Switch6/2
  main_cmd_duty_in/1 -> Switch6/3
  Constant11/1 -> Switch6/1
  Switch6/1 -> Switch1/2, [biprop_cmd_on]
  Constant1/1 -> Switch4/3
  desired_thrust/1 -> Switch4/1
  Switch4/1 -> csc_cac_coarse_acs_cntrl/8
  coarse_thr_descent/1 -> [coarse], Switch4/2
  Switch1/1 -> Bus Creator1/50, Gain1/1  "main_thruster_cmd"
  Bus Creator1/1 -> cnt_bus_msg/1
  quaternion_to_euler_angles (zyx)/1 -> Demux2/1
  quaternion_conjugate/1 -> quaternion_to_euler_angles (zyx)/1
  Demux2/1 -> [ppc_rotx_err]
  Demux2/3 -> [ppc_rotz_err]
  Demux2/2 -> [ppc_roty_err]
  enum_comparison/1 -> If/1
  If/1 -> csc_cac_coarse_acs_cntrl/Action
  If/2 -> csc_vac_vernier_acs_ctrl/Action
  Merge1/1 -> coarse_trq/1
  csc_cac_coarse_acs_cntrl/3 -> Merge1/1
  Merge2/1 -> verner_trq/1
  csc_cac_coarse_acs_cntrl/4 -> Merge2/1
  csc_vac_vernier_acs_ctrl/3 -> [vac_coarse_trq]
  [vac_coarse_trq] -> Merge1/2
  [vac_vernier_trq] -> Merge2/2
  cfe_tlm_header_align/1 -> Bus Creator1/1  "cfe_tlm_header_align"
  csc_vac_vernier_acs_ctrl/4 -> [vac_vernier_trq]
  csc_cac_coarse_acs_cntrl/2 -> Merge3/1
  Merge/1 -> Demux1/1
  Demux1/1 -> Bus Creator1/2  "coarse1_time"
  Demux1/8 -> Bus Creator1/9  "coarse8_time"
  Demux1/9 -> Bus Creator1/10  "coarse9_time"
  Demux1/12 -> Bus Creator1/13  "coarse12_time"
  Demux1/7 -> Bus Creator1/8  "coarse7_time"
  Demux1/4 -> Bus Creator1/5  "coarse4_time"
  Demux1/6 -> Bus Creator1/7  "coarse6_time"
  Demux1/3 -> Bus Creator1/4  "coarse3_time"
  Demux1/5 -> Bus Creator1/6  "coarse5_time"
  Demux1/10 -> Bus Creator1/11  "coarse10_time"
  Demux1/2 -> Bus Creator1/3  "coarse2_time"
  Demux1/11 -> Bus Creator1/12  "coarse11_time"
  Merge3/1 -> Demux4/1
  Demux5/3 -> Bus Creator1/16  "coarse3_delay"
  Demux5/4 -> Bus Creator1/17  "coarse4_delay"
  Demux5/6 -> Bus Creator1/19  "coarse6_delay"
  Demux5/8 -> Bus Creator1/21  "coarse8_delay"
  Demux5/2 -> Bus Creator1/15  "coarse2_delay"
  Demux5/12 -> Bus Creator1/25  "coarse12_delay"
  Demux5/9 -> Bus Creator1/22  "coarse9_delay"
  Demux5/5 -> Bus Creator1/18  "coarse5_delay"
  Demux5/1 -> Bus Creator1/14  "coarse1_delay"
  Demux5/11 -> Bus Creator1/24  "coarse11_delay"
  Demux5/7 -> Bus Creator1/20  "coarse7_delay"
  Demux5/10 -> Bus Creator1/23  "coarse10_delay"
  Demux4/4 -> Bus Creator1/29  "fine4_time"
  Demux4/9 -> Bus Creator1/34  "fine9_time"
  Demux4/10 -> Bus Creator1/35  "fine10_time"
  Demux4/8 -> Bus Creator1/33  "fine8_time"
  Demux4/7 -> Bus Creator1/32  "fine7_time"
  Demux4/2 -> Bus Creator1/27  "fine2_time"
  Demux4/1 -> Bus Creator1/26  "fine1_time"
  Demux4/5 -> Bus Creator1/30  "fine5_time"
  Demux4/12 -> Bus Creator1/37  "fine12_time"
  Demux4/3 -> Bus Creator1/28  "fine3_time"
  Demux4/6 -> Bus Creator1/31  "fine6_time"
  Demux4/11 -> Bus Creator1/36  "fine11_time"
  Constant4/1 -> Bus Creator1/53  "main_biprop_delay"
  Constant6/1 -> Bus Creator1/51  "main_thruster_delay"
  Demux6/1 -> Bus Creator1/38  "fine1_delay"
  Demux6/10 -> Bus Creator1/47  "fine10_delay"
  Demux6/4 -> Bus Creator1/41  "fine4_delay"
  Demux6/9 -> Bus Creator1/46  "fine9_delay"
  Demux6/6 -> Bus Creator1/43  "fine6_delay"
  Demux6/3 -> Bus Creator1/40  "fine3_delay"
  Demux6/8 -> Bus Creator1/45  "fine8_delay"
  Demux6/5 -> Bus Creator1/42  "fine5_delay"
  Demux6/2 -> Bus Creator1/39  "fine2_delay"
  Demux6/12 -> Bus Creator1/49  "fine12_delay"
  Demux6/7 -> Bus Creator1/44  "fine7_delay"
  Demux6/11 -> Bus Creator1/48  "fine11_delay"
  csc_vac_vernier_acs_ctrl/1 -> Merge3/2
  csc_vac_vernier_acs_ctrl/2 -> Merge/2
  Gain1/1 -> Bus Creator1/52  "main_biprop_monoprop"
  t_setting_roty_plus6/1 -> Demux5/1
  t_setting_roty_plus1/1 -> Demux6/1

== system mtv1_with_slosh_with_valve_delay/csci_gsse_mtv/csc_sim_mtv_simulation/create_sim_telem ==
  sim_data_bus : Inport
  time : Inport  Port=2
  Bus Creator : BusCreator  Inputs=9  OutDataTypeStr=Bus: sim_tlm_msg  NonVirtualBus=on
  Bus Selector2 : BusSelector  OutputSignals=lander_state_bus.rtk_pos_eci,lander_state_bus.rtk_vel_eci,lander_state_bus.rrk_q_body_from_eci,lander_state_bus.rtd_acc_body_in_eci,lander_state_bus.spacecraft_landed_flag,lander_state_bus.rrk_rate_body_eci_body,mass_props_msg.mass
  Gain : Gain
  Gain1 : Gain
  Terminator1 : Terminator
  Terminator2 : Terminator
  Terminator3 : Terminator
  byte_pad1 : util_common_lib/byte_pad  n_bytes=4
  cfe_tlm_header_align : util_common_lib/cfe_tlm_header_align
  kinematic_telemetry_conversion : telem_conversion_lib/kinematic_telemetry_conversion
  sim_tlm_msg : Outport
  wires:
  cfe_tlm_header_align/1 -> Bus Creator/1  "cfe_tlm_header_align"
  byte_pad1/1 -> Bus Creator/2  "pad1"
  kinematic_telemetry_conversion/3 -> Terminator3/1
  kinematic_telemetry_conversion/2 -> Terminator2/1
  kinematic_telemetry_conversion/1 -> Terminator1/1
  Bus Creator/1 -> sim_tlm_msg/1  "sim_tlm_msg"
  kinematic_telemetry_conversion/8 -> Bus Creator/7  "acc_topo"
  kinematic_telemetry_conversion/7 -> Bus Creator/6  "euler_zyx"
  kinematic_telemetry_conversion/6 -> Bus Creator/5  "q_topo_to_body"
  kinematic_telemetry_conversion/5 -> Bus Creator/4  "vel_topo"
  sim_data_bus/1 -> Bus Selector2/1
  time/1 -> kinematic_telemetry_conversion/1
  Bus Selector2/1 -> kinematic_telemetry_conversion/2  "<rtk_pos_eci>"
  Bus Selector2/2 -> kinematic_telemetry_conversion/3  "<rtk_vel_eci>"
  Bus Selector2/3 -> kinematic_telemetry_conversion/4  "<rrk_q_body_from_eci>"
  Bus Selector2/4 -> kinematic_telemetry_conversion/5  "<rtd_acc_body_in_eci>"
  Bus Selector2/6 -> Gain/1  "<rrk_rate_body_eci_body>"
  Gain/1 -> Bus Creator/8  "rate_body"
  Bus Selector2/7 -> Gain1/1  "<mass>"
  Gain1/1 -> Bus Creator/9  "mass"
  kinematic_telemetry_conversion/4 -> Bus Creator/3  "pos_topo"
  Bus Selector2/5 -> kinematic_telemetry_conversion/6  "<spacecraft_landed_flag>"

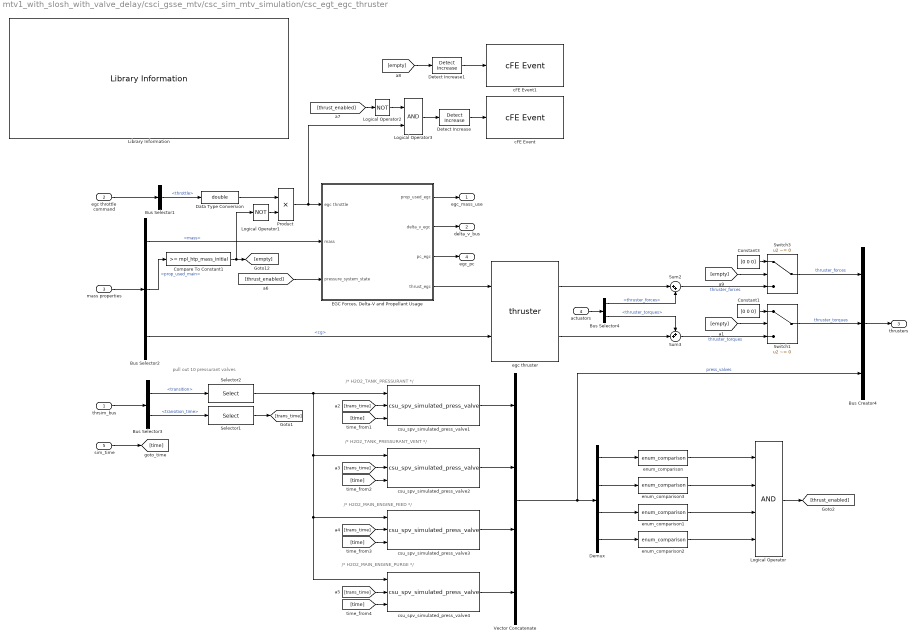
== system mtv1_with_slosh_with_valve_delay/csci_gsse_mtv/csc_sim_mtv_simulation/csc_egt_egc_thruster ==
  note: /* H2O2_MAIN_ENGINE_PURGE */
  note: /* H2O2_MAIN_ENGINE_FEED */
  note: /* H2O2_TANK_PRESSURANT_VENT */
  note: /* H2O2_TANK_PRESSURANT */
  note: pull out 10 pressurant valves
  thrsim_bus : Inport
  egc throttle command : Inport  Port=2
  mass properties : Inport  Port=3
  actuators : Inport  Port=4
  sim_time : Inport  Port=5
  Bus Creator4 : BusCreator  Inputs=3
  Bus Selector1 : BusSelector  OutputSignals=throttle
  Bus Selector2 : BusSelector  OutputSignals=mass,prop_used_main,cg
  Bus Selector3 : BusSelector  OutputSignals=transition,transition_time
  Bus Selector4 : BusSelector  OutputSignals=thruster_forces,thruster_torques
  Compare To Constant1 : simulink/Logic and Bit Operations/Compare To Constant  relop=>=  const=mpl_htp_mass_initial  OutDataTypeStr=boolean
  Constant1 : Constant  Value=[0 0 0]
  Constant3 : Constant  Value=[0 0 0]
  Data Type Conversion : DataTypeConversion  OutDataTypeStr=double
  Demux : Demux
  Detect Increase : simulink/Logic and Bit Operations/Detect Increase  vinit=0.0  InputProcessing=Inherited  OutDataTypeStr=boolean
  Detect Increase1 : simulink/Logic and Bit Operations/Detect Increase  vinit=0.0  InputProcessing=Inherited  OutDataTypeStr=boolean
  "EGC Forces, Delta-V and Propellant Usage" : Subsystem
  Library Information : util_info_lib/Library Information  owner='NONE'
  Logical Operator : Logic  Inputs=4  AllPortsSameDT=off  OutDataTypeStr=boolean
  Logical Operator1 : Logic  Operator=NOT  AllPortsSameDT=off  OutDataTypeStr=boolean
  Logical Operator2 : Logic  Operator=NOT  AllPortsSameDT=off  OutDataTypeStr=boolean
  Logical Operator3 : Logic  AllPortsSameDT=off  OutDataTypeStr=boolean
  Product : Product
  Selector1 : Selector  InputPortWidth=22  Indices=[13:22]
  Selector2 : Selector  InputPortWidth=22  Indices=[13:22]
  Sum2 : Sum  Inputs=|++
  Sum3 : Sum  Inputs=++|
  Switch1 : Switch  Criteria=u2 ~= 0
  Switch3 : Switch  Criteria=u2 ~= 0
  Vector Concatenate : Concatenate  NumInputs=4
  cFE Event : util_event_lib/cFE Event  event_message='EGC commanded with bad latch valve config. No thrust.'  event_id=22  event_severity=INFORMATION  event_use_enums=off  event_enum_types={}
  cFE Event1 : util_event_lib/cFE Event  event_message='Out of HTP!'  event_id=22  event_severity=INFORMATION  event_use_enums=off  event_enum_types={}
  csu_spv_simulated_press_valve1 : csu_spv_simulated_press_valves_lib/csu_spv_simulated_press_valve  thruster_idx=1  num_thrusters=10  energized_value=1  deenergized_value=0
  csu_spv_simulated_press_valve2 : csu_spv_simulated_press_valves_lib/csu_spv_simulated_press_valve  thruster_idx=2  num_thrusters=10  energized_value=0  deenergized_value=1
  csu_spv_simulated_press_valve3 : csu_spv_simulated_press_valves_lib/csu_spv_simulated_press_valve  thruster_idx=4  num_thrusters=10  energized_value=1  deenergized_value=0
  csu_spv_simulated_press_valve4 : csu_spv_simulated_press_valves_lib/csu_spv_simulated_press_valve  thruster_idx=5  num_thrusters=10  energized_value=1  deenergized_value=0
  egc thruster : util_thruster_lib/thruster  Thruster_Position=tfl_thruster_egc_position  Thruster_Orientation=tfl_thruster_egc_orientation
  enum_comparison{,1..3} (4 alike) : util_common_lib/enum_comparison  comparison_type===
  egc_mass_use : Outport
  delta_v_bus : Outport  Port=2
  thrusters : Outport  Port=3
  egc_pc : Outport  Port=4
  wires:
  "EGC Forces, Delta-V and Propellant Usage"/3(pc_egc) -> egc_pc/1
  Product/1 -> Logical Operator3/2, "EGC Forces, Delta-V and Propellant Usage"/1(egc throttle)
  Switch1/1 -> Bus Creator4/2  "thruster_torques"
  Switch3/1 -> Bus Creator4/1  "thruster_forces"
  Constant3/1 -> Switch3/1
  egc throttle command/1 -> Bus Selector1/1
  Data Type Conversion/1 -> Product/1
  Sum2/1 -> Switch3/3  "thruster_forces"
  Sum3/1 -> Switch1/3  "thruster_torques"
  Bus Creator4/1 -> thrusters/1
  Bus Selector4/2 -> Sum3/1  "<thruster_torques>"
  egc thruster/2 -> Sum3/2
  egc thruster/1 -> Sum2/1
  actuators/1 -> Bus Selector4/1
  Bus Selector4/1 -> Sum2/2  "<thruster_forces>"
  Bus Selector2/3 -> egc thruster/2  "<cg>"
  Bus Selector2/1 -> "EGC Forces, Delta-V and Propellant Usage"/2(mass)  "<mass>"
  mass properties/1 -> Bus Selector2/1
  "EGC Forces, Delta-V and Propellant Usage"/4(thrust_egc) -> egc thruster/1
  "EGC Forces, Delta-V and Propellant Usage"/2(delta_v_egc) -> delta_v_bus/1
  "EGC Forces, Delta-V and Propellant Usage"/1(prop_used_egc) -> egc_mass_use/1
  Bus Selector1/1 -> Data Type Conversion/1  "<throttle>"
  Constant1/1 -> Switch1/1
  Compare To Constant1/1 -> [empty], Logical Operator1/1
  [empty] -> Switch3/2
  [empty] -> Switch1/2
  thrsim_bus/1 -> Bus Selector3/1
  Selector1/1 -> [trans_time]
  Bus Selector3/1 -> Selector2/1  "<transition>"
  Bus Selector3/2 -> Selector1/1  "<transition_time>"
  [trans_time] -> csu_spv_simulated_press_valve1/2
  sim_time/1 -> [time]
  [time] -> csu_spv_simulated_press_valve1/3
  [trans_time] -> csu_spv_simulated_press_valve2/2
  [time] -> csu_spv_simulated_press_valve2/3
  [trans_time] -> csu_spv_simulated_press_valve3/2
  [time] -> csu_spv_simulated_press_valve3/3
  [trans_time] -> csu_spv_simulated_press_valve4/2
  [time] -> csu_spv_simulated_press_valve4/3
  Selector2/1 -> csu_spv_simulated_press_valve4/1, csu_spv_simulated_press_valve3/1, csu_spv_simulated_press_valve2/1, csu_spv_simulated_press_valve1/1
  csu_spv_simulated_press_valve1/1 -> Vector Concatenate/1
  csu_spv_simulated_press_valve3/1 -> Vector Concatenate/3
  csu_spv_simulated_press_valve4/1 -> Vector Concatenate/4
  csu_spv_simulated_press_valve2/1 -> Vector Concatenate/2
  enum_comparison/1 -> Logical Operator/1
  enum_comparison3/1 -> Logical Operator/2
  enum_comparison1/1 -> Logical Operator/3
  enum_comparison2/1 -> Logical Operator/4
  Logical Operator/1 -> [thrust_enabled]
  [thrust_enabled] -> "EGC Forces, Delta-V and Propellant Usage"/3(pressure_system_state)
  Bus Selector2/2 -> Compare To Constant1/1  "<prop_used_main>"
  Logical Operator1/1 -> Product/2
  Vector Concatenate/1 -> Bus Creator4/3, Demux/1  "press_valves"
  Demux/1 -> enum_comparison/1
  Demux/2 -> enum_comparison3/1
  Demux/3 -> enum_comparison1/1
  Demux/4 -> enum_comparison2/1
  Logical Operator3/1 -> Detect Increase/1
  Logical Operator2/1 -> Logical Operator3/1
  [thrust_enabled] -> Logical Operator2/1
  Detect Increase/1 -> cFE Event/1
  [empty] -> Detect Increase1/1
  Detect Increase1/1 -> cFE Event1/1
